simulink model "control"  (R2024b)
settings: Solver=VariableStepAuto  StartTime=0.0  StopTime=3  RelTol=1e-3
settings Model: Creator=usuario  LastModifiedBy=usuario

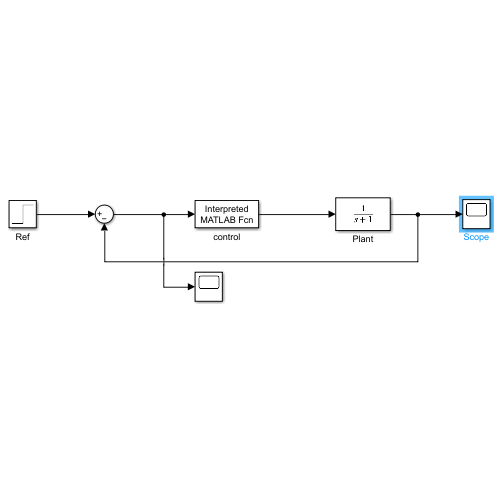
[thumbnail: Simulink's stored preview of the top-level diagram]
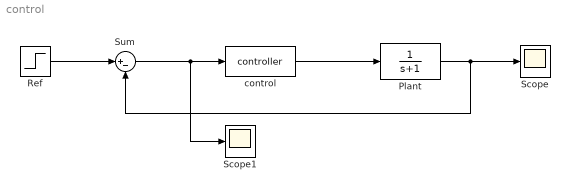
== system control ==
  Plant : TransferFcn  Denominator=[1 1]
  Ref : Step  SampleTime=0
  Scope : Scope
  Scope1 : Scope
  Sum : Sum  Inputs=|+-
  control : MATLABFcn  MATLABFcn=controller
  wires:
  Sum/1 -> Scope1/1, control/1
  control/1 -> Plant/1
  Plant/1 -> Sum/2, Scope/1
  Ref/1 -> Sum/1
